simulink model "exp11_6"  (R2019b)
settings: Solver=FixedStepAuto  StartTime=0.0  StopTime=5  FixedStep=0.01  RelTol=1e-3
settings Model: Creator=Sing Ngai  LastModifiedBy=Sing Ngai

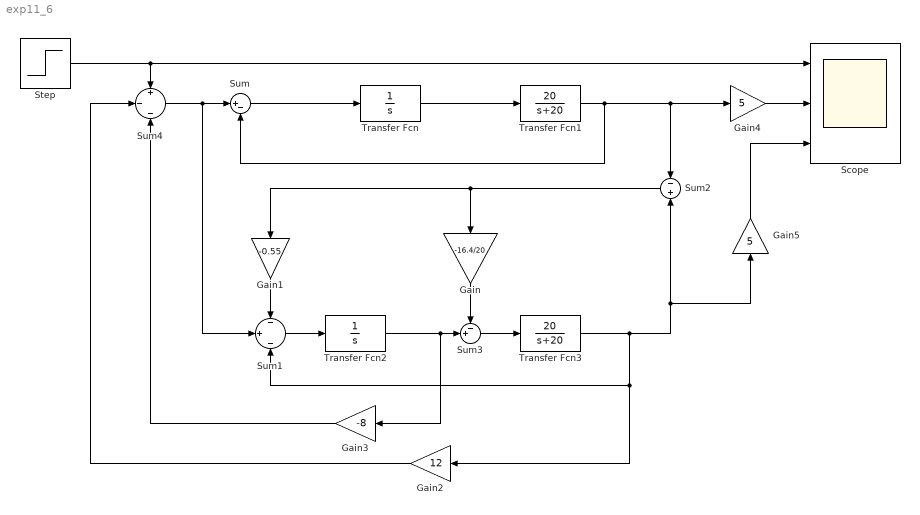
== system exp11_6 ==
  Gain : Gain  Gain=-16.4/20
  Gain1 : Gain  Gain=-0.55
  Gain2 : Gain  Gain=12
  Gain3 : Gain  Gain=-8
  Gain4 : Gain  Gain=5
  Gain5 : Gain  Gain=5
  Scope : Scope  NumInputPorts=3
  Step : Step  Before=1  SampleTime=0
  Sum : Sum  Inputs=|+-
  Sum1 : Sum  Inputs=-|+|-
  Sum2 : Sum  Inputs=-|+
  Sum3 : Sum  Inputs=-+|
  Sum4 : Sum  Inputs=+|-|-
  Transfer Fcn : TransferFcn  Denominator=[1 0]
  Transfer Fcn1 : TransferFcn  Numerator=[20]  Denominator=[1 20]
  Transfer Fcn2 : TransferFcn  Denominator=[1 0]
  Transfer Fcn3 : TransferFcn  Numerator=[20]  Denominator=[1 20]
  wires:
  Transfer Fcn/1 -> Transfer Fcn1/1
  Sum/1 -> Transfer Fcn/1
  Sum1/1 -> Transfer Fcn2/1
  Transfer Fcn1/1 -> Sum/2, Sum2/1, Gain4/1
  Transfer Fcn3/1 -> Sum1/3, Gain2/1, Gain5/1, Sum2/2
  Sum2/1 -> Gain1/1, Gain/1
  Gain1/1 -> Sum1/1
  Sum3/1 -> Transfer Fcn3/1
  Gain/1 -> Sum3/1
  Transfer Fcn2/1 -> Gain3/1, Sum3/2
  Step/1 -> Sum4/1, Scope/1
  Sum4/1 -> Sum1/2, Sum/1
  Gain3/1 -> Sum4/3
  Gain2/1 -> Sum4/2
  Gain4/1 -> Scope/2
  Gain5/1 -> Scope/3
